simulink model "BuckTest"  (R2025a)
settings: Solver=VariableStepAuto  StartTime=0.0  StopTime=1  RelTol=1e-3
values from neighbouring files (symbols this model uses):
  A = [-(Rl + D_prime * Rp_ac)/L ,          -(D_prime * R_ac)/(L * R_sum_ac) ... (first row only)    [BoostSS.m]    (also in BoostSS_Input.m = [ 0            ,  1/L              , -D_prime/L; BuckSS.m = [-((Rl + (Rload * Rc_eqv)/R_sum)/L)  ,   -(Rload / (L * R_su; BuckSS_Input.m = [ 0            ,  Duty/L           , -1/L)
  B = [ (Rp_ac * I_L + (R_ac * V_C)/R_sum_ac)/L ,  0 ... (first row only)    [BoostSS.m]    (also in BoostSS_Input.m = [ V_Co/L; BuckSS.m = [Vin/L ,     0; BuckSS_Input.m = [ V_Cin/L)
  C = [ D_prime * Rp_ac, R_ac/R_sum_ac ... (first row only)    [BoostSS.m]    (also in BuckSS.m = [(Rload * Rc_eqv)/R_sum , Rload/R_sum)
  D = [ -Rp_ac * I_L   , 0 ... (first row only)    [BoostSS.m]    (also in BuckSS.m = [0, 0)
  gm = 250e-6    (= 0.00025)    [BoostSS.m]    (also in BoostSS_Input.m; BuckSS.m; BuckSS_Input.m)
settings Model: Creator=lebla  LastModifiedBy=lebla

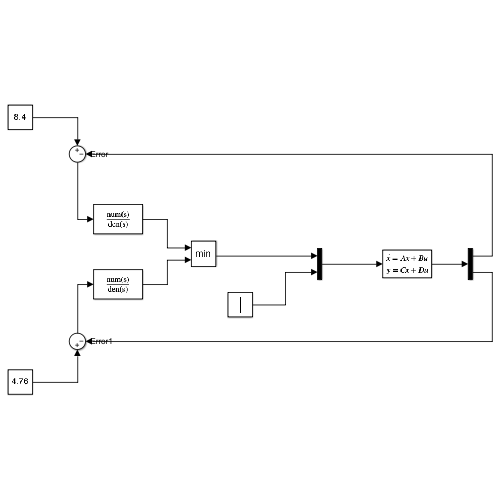
[thumbnail: Simulink's stored preview of the top-level diagram]
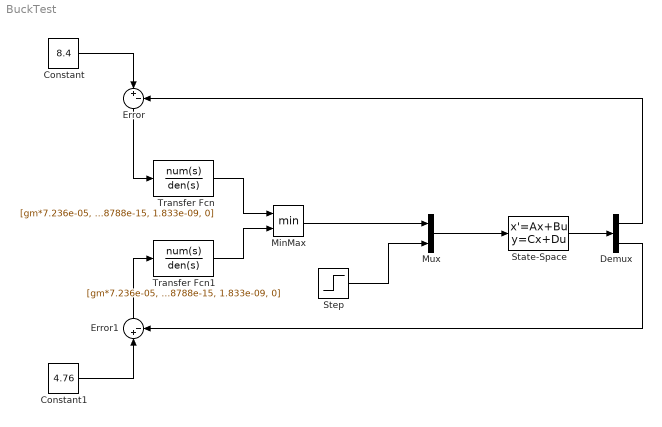
== system BuckTest ==
  Constant : Constant  Value=8.4
  Constant1 : Constant  Value=4.76
  Demux : Demux  Outputs=2
  Error : Sum  Inputs=|+-
  Error1 : Sum  Inputs=|+-
  MinMax : MinMax  Inputs=2
  Mux : Mux  Inputs=2
  State-Space : StateSpace  A=A  B=B  C=C  D=D  InitialCondition=0
  Step : Step  Time=0.01  After=5  SampleTime=0
  Transfer Fcn : TransferFcn  Numerator=[gm*7.236e-05, gm]  Denominator=[2.38788e-15, 1.833e-09, 0]
  Transfer Fcn1 : TransferFcn  Numerator=[gm*7.236e-05, gm]  Denominator=[2.38788e-15, 1.833e-09, 0]
  wires:
  Mux/1 -> State-Space/1
  Step/1 -> Mux/2
  Constant/1 -> Error/1
  State-Space/1 -> Demux/1
  Demux/1 -> Error/2
  Constant1/1 -> Error1/1
  Demux/2 -> Error1/2
  MinMax/1 -> Mux/1
  Transfer Fcn1/1 -> MinMax/2
  Transfer Fcn/1 -> MinMax/1
  Error1/1 -> Transfer Fcn1/1
  Error/1 -> Transfer Fcn/1
